simulink model "TBS_SIM_UDP_HIL"  (R2016b)
settings: Solver=ode5  StartTime=0.0  StopTime=inf  FixedStep=0.005  RelTol=1e-3  EnableMultiTasking=on
PreLoadFcn:
  | TBS_Cai_simu_init_20170316
StopFcn:
  | TBS_SIMULATION_LOG
undefined symbols (not defined in the file): air_density, L1X, L2X, L3X, L3Y, MAC1, MAC2, MAC3, magnitude, motor_m0, motor_t0, ORIGIN_CD, ORIGIN_CL, ORIGIN_CM, S_seg1, S_seg2, S_seg3, Standard_Devices, UDP_Protocol, y_ac
libraries: aerolibconvert2 x9, sldrtlib x4, aerolibwind2 x3, aerolibtransform2 x2, aerolib6dof2 x1, simulink x1, aerolibasang x1
settings Model: SimulationMode=external  Creator=SUN Jingxuan  LastModifiedBy=SUN Jingxuan
settings SolverCC: EnableConcurrentExecution=on
settings DataIOCC: LimitDataPoints=on  SaveFormat=StructureWithTime
settings OptimizationCC: BlockReduction=off  OptimizeBlockIOStorage=off  BufferReuse=off  GlobalBufferReuse=off  ExpressionFolding=off  LocalBlockOutputs=off
settings DebuggingCC: SFUnexpectedBacktrackingDiag=warning  SFNoUnconditionalDefaultTransitionDiag=warning  SFExecutionAtInitializationDiag=none
settings HardwareCC: TargetBitPerLong=64  TargetBitPerPointer=64  TargetIntDivRoundTo=Zero  TargetEndianess=LittleEndian  TargetWordSize=64  TargetHWDeviceType=Intel->x86-64
settings ModelReferenceCC: PropagateSignalLabelsOutOfModel=off
settings RTWCC: SystemTargetFile=sldrt.tlc  TemplateMakefile=sldrt.tmf  Description=Simulink Desktop Real-Time  RTWCompilerOptimization=on
settings CodeAppCC: MaxIdLength=95
settings SimulinkDesktopRealTimeCC: TargetPreCompLibLocation=E:\MATLAB2016\toolbox\sldrt\lib\win64  TargetLangStandard=C89/C90 (ANSI)  SupportVariableSizeSignals=off
settings ConfigComp: CovMetricSettings=dw  CovHtmlReporting=on  CovSaveCumulativeToWorkspaceVar=on  CovSaveSingleToWorkspaceVar=on  CovExternalEMLEnable=off

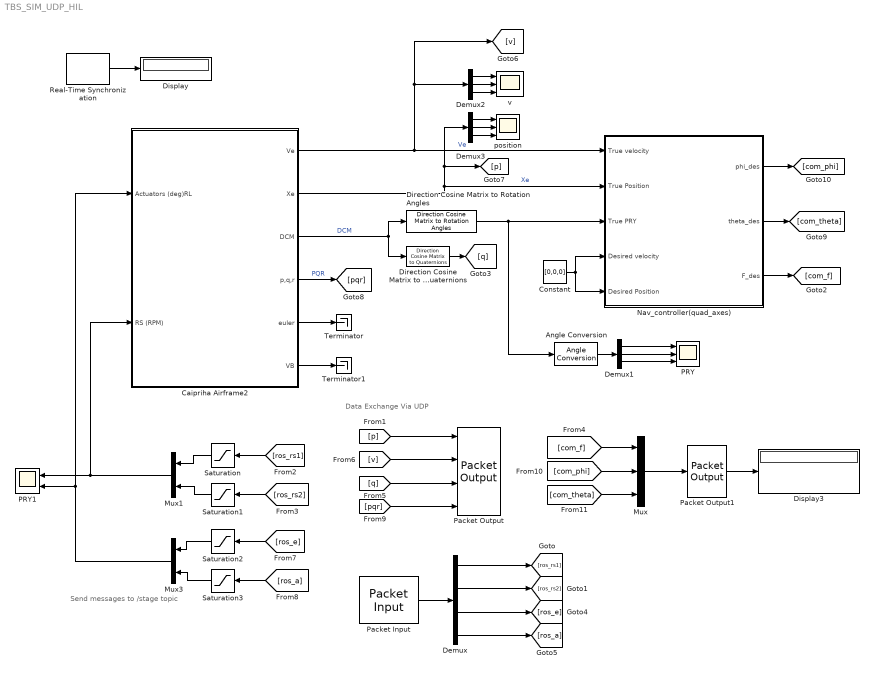
== system TBS_SIM_UDP_HIL ==
  note: Data Exchange Via UDP
  note: Send messages to /stage topic
  Angle Conversion : aerolibconvert2/Angle Conversion  IU=rad  OU=deg
  Caipriha Airframe2 : Subsystem
  Constant : Constant  Value=[0,0,0]
  Demux : Demux
  Demux1 : Demux  Outputs=3
  Demux2 : Demux  Outputs=3
  Demux3 : Demux  Outputs=3
  Direction Cosine Matrix to Rotation Angles : aerolibtransform2/Direction Cosine Matrix to Rotation Angles  rotationOrder=YZX  lim=Default
      settings: AttributesFormatString=Rotation Order: %<rotationOrder>
  Direction Cosine Matrix to Quaternions : aerolibtransform2/Direction Cosine Matrix  to Quaternions
  Display : Display
  Display3 : Display
  Mux : Mux  Inputs=3
  Mux1 : Mux  Inputs=2
  Mux3 : Mux  Inputs=2
  Nav_controller(quad_axes) : Subsystem
  PRY : Scope  NumInputPorts=3
  PRY1 : Scope  NumInputPorts=2
  Packet Input : sldrtlib/Packet Input  SampleTime=-1  MaxMissedTicks=10  ShowMissedTicks=off  YieldWhenWaiting=off  DrvName=Standard_Devices/UDP_Protocol  DrvAddress=49001  DrvOptions=[3232235791 49001]  PacketSize=32  DataTypes='4*double'  ShowReady=off  ShowError=off  PacketID=1  ByteOrder=1  ShowTimestamp=off
      settings: AttributesFormatString=Standard Devices\nUDP Protocol [BF69h]
  Packet Output : sldrtlib/Packet Output  SampleTime=-1  MaxMissedTicks=10  ShowMissedTicks=off  YieldWhenWaiting=off  DrvName=Standard_Devices/UDP_Protocol  DrvAddress=49005  DrvOptions=[3232235791 49000]  PacketSize=104  DataTypes={'3*double','3*double','4*double','3*double'}  ShowReady=off  ShowError=off  PacketID=1  ByteOrder=1  InitialValue=[0 0 0 0 0 0 0.7071 0 -0.7071 0 0 0 0]  FinalValue=[]
      settings: AttributesFormatString=Standard Devices\nUDP Protocol [BF6Dh]
  Packet Output1 : sldrtlib/Packet Output  SampleTime=-1  MaxMissedTicks=10  ShowMissedTicks=on  YieldWhenWaiting=off  DrvName=Standard_Devices/UDP_Protocol  DrvAddress=49006  DrvOptions=[3232235791 49005]  PacketSize=24  DataTypes='3*double'  ShowReady=off  ShowError=off  PacketID=1  ByteOrder=1  InitialValue=[8;0;0]  FinalValue=[]
      settings: AttributesFormatString=Standard Devices\nUDP Protocol [BF6Eh]
  Real-Time Synchronization : sldrtlib/Real-Time Synchronization  SampleTime=0.02  MaxMissedTicks=10  ShowMissedTicks=on  YieldWhenWaiting=off
  Saturation : Saturate  UpperLimit=10000  LowerLimit=0
  Saturation1 : Saturate  UpperLimit=10000  LowerLimit=0
  Saturation2 : Saturate  UpperLimit=16.5  LowerLimit=-23
  Saturation3 : Saturate  UpperLimit=16.5  LowerLimit=-23
  Terminator : Terminator
  Terminator1 : Terminator
  position : Scope  NumInputPorts=3
  "v " : Scope  NumInputPorts=3
  wires:
  Mux3/1 -> Caipriha Airframe2/1(Actuators (deg)RL), PRY1/2
  Mux1/1 -> Caipriha Airframe2/2(RS (RPM)), PRY1/1
  Constant/1 -> Nav_controller(quad_axes)/4(Desired velocity), Nav_controller(quad_axes)/5(Desired Position)
  Saturation/1 -> Mux1/1
  Saturation1/1 -> Mux1/2
  Saturation2/1 -> Mux3/1
  Saturation3/1 -> Mux3/2
  Demux2/1 -> "v "/1
  Demux2/2 -> "v "/2
  Demux2/3 -> "v "/3
  Caipriha Airframe2/1(Ve) -> [v], Demux2/1, Nav_controller(quad_axes)/1(True velocity)  "Ve"
  Demux3/1 -> position/1
  Demux3/2 -> position/2
  Demux3/3 -> position/3
  Caipriha Airframe2/2(Xe) -> Demux3/1, [p], Nav_controller(quad_axes)/2(True Position)  "Xe"
  Caipriha Airframe2/3(DCM) -> Direction Cosine Matrix to Rotation Angles/1, Direction Cosine Matrix to Quaternions/1  "DCM"
  Direction Cosine Matrix to Rotation Angles/1 -> Angle Conversion/1, Nav_controller(quad_axes)/3(True PRY)
  Demux1/1 -> PRY/1
  Demux1/2 -> PRY/2
  Demux1/3 -> PRY/3
  Angle Conversion/1 -> Demux1/1
  Nav_controller(quad_axes)/3(F_des) -> [com_f]
  Nav_controller(quad_axes)/2("theta_des ") -> [com_theta]
  Nav_controller(quad_axes)/1(phi_des) -> [com_phi]
  [ros_rs1] -> Saturation/1
  [ros_rs2] -> Saturation1/1
  [ros_e] -> Saturation2/1
  [ros_a] -> Saturation3/1
  Direction Cosine Matrix to Quaternions/1 -> [q]
  [p] -> Packet Output/1
  [pqr] -> Packet Output/4
  [v] -> Packet Output/2
  [q] -> Packet Output/3
  Packet Input/1 -> Demux/1
  Demux/1 -> [ros_rs1]
  Demux/2 -> [ros_rs2]
  Demux/3 -> [ros_e]
  Demux/4 -> [ros_a]
  Mux/1 -> Packet Output1/1
  Packet Output1/1 -> Display3/1
  Real-Time Synchronization/1 -> Display/1
  Caipriha Airframe2/4(p,q,r) -> [pqr]  "PQR"
  [com_f] -> Mux/1
  [com_phi] -> Mux/2
  [com_theta] -> Mux/3
  Caipriha Airframe2/5(euler) -> Terminator/1
  Caipriha Airframe2/6("VB ") -> Terminator1/1

== system TBS_SIM_UDP_HIL/Caipriha Airframe2 ==
  Actuators (deg)RL : Inport
  RS (RPM) : Inport  Port=2
  6DOF (Quaternion) : aerolib6dof2/6DOF (Euler Angles)  units=Metric (MKS)  mtype=Fixed  rep=Quaternion  xme_0=init_pos_hov  Vm_0=init_vel_hov  eul_0=init_att_hov  pm_0=[0 0 0]  mass_0=0.876  mass_e=0.5  mass_f=2.0  inertia=Inertia  inertia_e=eye(3)  inertia_f=2*eye(3)  k_quat=1.0  vre_flag=on
  Aerodynamic Coefficient : Subsystem
  Alpha,Beta,Mach : Subsystem  AncestorBlock=aeroblk_lib_HL20/HL20 Airframe/Alpha,Beta,Mach
  Angle Conversion : aerolibconvert2/Angle Conversion  IU=rad  OU=deg
  Constant2 : Constant  Value=8.541
  Display2 : Display
  Environment Models1 : Subsystem  AncestorBlock=aeroblk_lib_HL20/HL20 Airframe/Environment Models
  Force&Moments : Subsystem
  Scope : Scope
  Terminator1 : Terminator  Commented=on
  Terminator2 : Terminator  Commented=on
  "Thrust " : Subsystem
  Ve : Outport  InitialOutput=0
  Xe : Outport  Port=2  InitialOutput=0
  DCM : Outport  Port=3  InitialOutput=0
  p,q,r : Outport  Port=4  InitialOutput=0
  euler : Outport  Port=5  InitialOutput=0
  "VB " : Outport  Port=6  InitialOutput=0
  wires:
  6DOF (Quaternion)/5 -> "VB "/1, Alpha,Beta,Mach/2(Vb)
  6DOF (Quaternion)/1 -> Environment Models1/1(Ve), Ve/1
  Constant2/1 -> Force&Moments/5(Gravity)
  6DOF (Quaternion)/4 -> Environment Models1/3(DCM), DCM/1, Force&Moments/6(DCM)
  6DOF (Quaternion)/3 -> euler/1
  Alpha,Beta,Mach/3(V_aircraft) -> Aerodynamic Coefficient/4(V), "Thrust "/2("AS ")
  Alpha,Beta,Mach/2(Incid) -> Angle Conversion/1, Aerodynamic Coefficient/5(Incid)
  "Thrust "/2(MT1) -> Force&Moments/2(MT)
  "Thrust "/1(F_T) -> Force&Moments/1("FT ")
  "Thrust "/4(T2) -> Aerodynamic Coefficient/2(T2)
  "Thrust "/3(T1) -> Aerodynamic Coefficient/1("T1 ")
  Aerodynamic Coefficient/2(M) -> Force&Moments/4(M)
  Aerodynamic Coefficient/1(F) -> Force&Moments/3(F)
  RS (RPM)/1 -> "Thrust "/1(RS1)
  Actuators (deg)RL/1 -> Aerodynamic Coefficient/3(Actuators)
  Environment Models1/1(Wind Velocity) -> Alpha,Beta,Mach/1(Wind Velocity)
  6DOF (Quaternion)/7 -> Terminator2/1
  6DOF (Quaternion)/6 -> p,q,r/1
  6DOF (Quaternion)/2 -> Environment Models1/2(Position), Xe/1
  6DOF (Quaternion)/8 -> Terminator1/1
  Force&Moments/2(LMN) -> 6DOF (Quaternion)/2
  Force&Moments/1(X,Y,Z) -> 6DOF (Quaternion)/1
  Alpha,Beta,Mach/1("[Vb]_total") -> Aerodynamic Coefficient/6(Vb_total)
  Angle Conversion/1 -> Scope/1, Display2/1

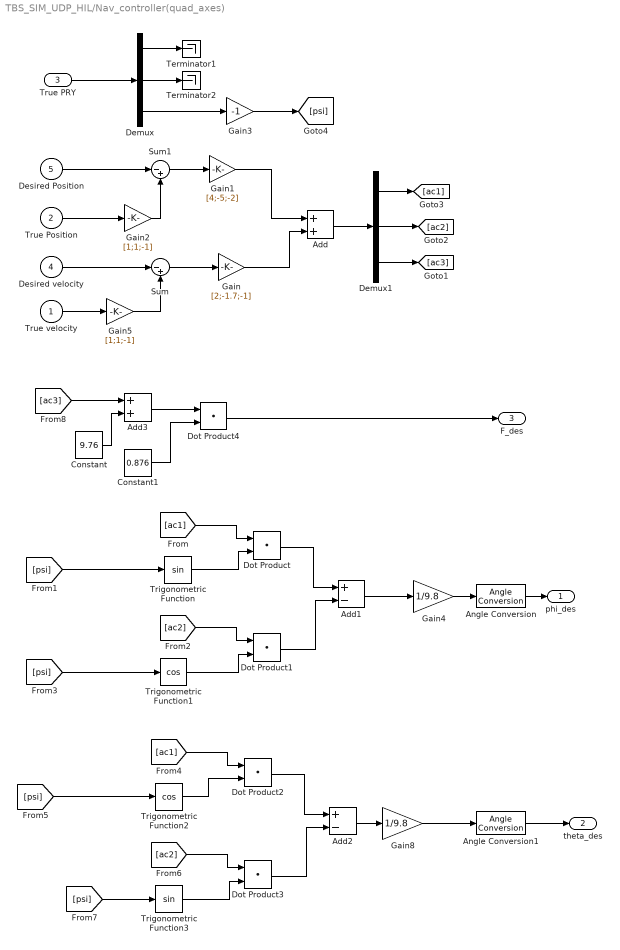
== system TBS_SIM_UDP_HIL/Nav_controller(quad_axes) ==
  True velocity : Inport
  True Position : Inport  Port=2
  True PRY : Inport  Port=3
  Desired velocity : Inport  Port=4
  Desired Position : Inport  Port=5
  Add : Sum
  Add1 : Sum  Inputs=+-
  Add2 : Sum  Inputs=+-
  Add3 : Sum
  Angle Conversion : aerolibconvert2/Angle Conversion  IU=rad  OU=deg
  Angle Conversion1 : aerolibconvert2/Angle Conversion  IU=rad  OU=deg
  Constant : Constant  Value=9.76
  Constant1 : Constant  Value=0.876
  Demux : Demux  Outputs=3
  Demux1 : Demux  Outputs=3
  Dot Product{,1..4} (5 alike) : DotProduct  InputSameDT=on  OutDataTypeStr=Inherit: Inherit via internal rule
  Gain : Gain  Gain=[2;-1.7;-1]
  Gain1 : Gain  Gain=[4;-5;-2]
  Gain2 : Gain  Gain=[1;1;-1]
  Gain3 : Gain  Gain=-1
  Gain4 : Gain  Gain=1/9.8
  Gain5 : Gain  Gain=[1;1;-1]
  Gain8 : Gain  Gain=1/9.8
  Sum : Sum  Inputs=|-+
  Sum1 : Sum  Inputs=|-+
  Terminator1 : Terminator
  Terminator2 : Terminator
  Trigonometric Function : Trigonometry
  Trigonometric Function1 : Trigonometry  Operator=cos
  Trigonometric Function2 : Trigonometry  Operator=cos
  Trigonometric Function3 : Trigonometry
  phi_des : Outport
  "theta_des " : Outport  Port=2
  F_des : Outport  Port=3
  wires:
  True velocity/1 -> Gain5/1
  Desired velocity/1 -> Sum/1
  Sum/1 -> Gain/1
  Sum1/1 -> Gain1/1
  Gain1/1 -> Add/1
  Gain/1 -> Add/2
  True PRY/1 -> Demux/1
  Demux/1 -> Terminator1/1
  Demux/3 -> Gain3/1
  Demux/2 -> Terminator2/1
  Add/1 -> Demux1/1
  Demux1/2 -> [ac2]
  [ac1] -> Dot Product/1
  Trigonometric Function/1 -> Dot Product/2
  [psi] -> Trigonometric Function/1
  [ac2] -> Dot Product1/1
  Trigonometric Function1/1 -> Dot Product1/2
  [psi] -> Trigonometric Function1/1
  Dot Product/1 -> Add1/1
  Dot Product1/1 -> Add1/2
  Add1/1 -> Gain4/1
  [ac1] -> Dot Product2/1
  Trigonometric Function2/1 -> Dot Product2/2
  [psi] -> Trigonometric Function2/1
  [ac2] -> Dot Product3/1
  Trigonometric Function3/1 -> Dot Product3/2
  [psi] -> Trigonometric Function3/1
  Dot Product2/1 -> Add2/1
  Dot Product3/1 -> Add2/2
  Add2/1 -> Gain8/1
  [ac3] -> Add3/1
  Constant/1 -> Add3/2
  Add3/1 -> Dot Product4/1
  Constant1/1 -> Dot Product4/2
  Dot Product4/1 -> F_des/1
  Demux1/1 -> [ac1]
  Demux1/3 -> [ac3]
  True Position/1 -> Gain2/1
  Gain2/1 -> Sum1/2
  Desired Position/1 -> Sum1/1
  Gain3/1 -> [psi]
  Gain4/1 -> Angle Conversion/1
  Angle Conversion/1 -> phi_des/1
  Gain8/1 -> Angle Conversion1/1
  Angle Conversion1/1 -> "theta_des "/1
  Gain5/1 -> Sum/2

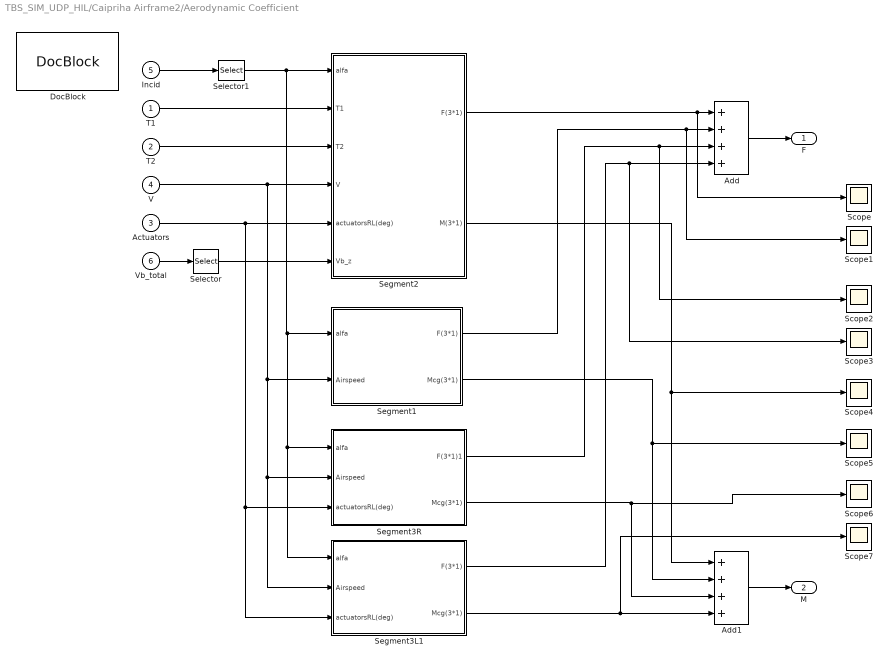
== system TBS_SIM_UDP_HIL/Caipriha Airframe2/Aerodynamic Coefficient ==
  "T1 " : Inport
  T2 : Inport  Port=2
  Actuators : Inport  Port=3
  V : Inport  Port=4
  Incid : Inport  Port=5
  Vb_total : Inport  Port=6
  Add : Sum  Inputs=++++
  Add1 : Sum  Inputs=++++
  DocBlock : simulink/Model-Wide Utilities/DocBlock  DocumentType=Text
      content=|
      | Segment definition: F:\MATLAB\TBS dynamic\segment.png
  Scope{,1..7} (8 alike) : Scope
  Segment1 : Subsystem
  Segment2 : Subsystem
  Segment3L1 : Subsystem
  Segment3R : Subsystem
  Selector : Selector  InputPortWidth=3  IndexOptions=Index vector (dialog)  Indices=[3]  OutputSizes=1
  Selector1 : Selector  InputPortWidth=2  IndexOptions=Index vector (dialog)  Indices=[1]  OutputSizes=1
  F : Outport
  M : Outport  Port=2
  wires:
  T2/1 -> Segment2/3(T2)
  "T1 "/1 -> Segment2/2("T1 ")
  Selector1/1 -> Segment3L1/1(alfa), Segment3R/1(alfa), Segment1/1(alfa), Segment2/1(alfa)
  Incid/1 -> Selector1/1
  Actuators/1 -> Segment3L1/3("actuatorsRL(deg) "), Segment3R/3("actuatorsRL(deg) "), Segment2/5("actuatorsRL(deg) ")
  V/1 -> Segment3L1/2(Airspeed), Segment3R/2(Airspeed), Segment1/2(Airspeed), Segment2/4(V)
  Selector/1 -> Segment2/6(Vb_z)
  Vb_total/1 -> Selector/1
  Segment2/1(F(3*1)) -> Scope/1, Add/1
  Segment1/1(F(3*1)) -> Scope1/1, Add/2
  Segment3R/1(F(3*1)1) -> Add/3, Scope2/1
  Segment3L1/1(F(3*1)) -> Scope3/1, Add/4
  Add/1 -> F/1
  Add1/1 -> M/1
  Segment2/2(M(3*1)) -> Scope4/1, Add1/1
  Segment1/2(Mcg(3*1)) -> Add1/2, Scope5/1
  Segment3R/2(Mcg(3*1)) -> Scope6/1, Add1/3
  Segment3L1/2(Mcg(3*1)) -> Scope7/1, Add1/4

== system TBS_SIM_UDP_HIL/Caipriha Airframe2/Alpha,Beta,Mach ==
  Wind Velocity : Inport  PortDimensions=3
  Vb : Inport  Port=2  PortDimensions=3
  "Incidence, Sideslip & Airspeed" : aerolibasang/Incidence, Sideslip, & Airspeed
  Mux : Mux  Inputs=2
  Sum : Sum  Inputs=|+-  SaturateOnIntegerOverflow=on  InputSameDT=on  OutDataTypeStr=Inherit: Same as first input
  "[Vb]_total" : Outport
  Incid : Outport  Port=2
  V_aircraft : Outport  Port=3
  wires:
  Sum/1 -> "[Vb]_total"/1, "Incidence, Sideslip & Airspeed"/1
  Wind Velocity/1 -> Sum/2
  "Incidence, Sideslip & Airspeed"/1 -> Mux/1  "Alpha"
  Mux/1 -> Incid/1
  "Incidence, Sideslip & Airspeed"/2 -> Mux/2  "Beta"
  Vb/1 -> Sum/1
  "Incidence, Sideslip & Airspeed"/3 -> V_aircraft/1

== system TBS_SIM_UDP_HIL/Caipriha Airframe2/Environment Models1 ==
  Ve : Inport
  Position : Inport  Port=2
  DCM : Inport  Port=3
  Abs : Abs
  Discrete Wind Gust Model : aerolibwind2/Discrete Wind Gust Model  units=Metric (MKS)  Gx=on  Gy=on  Gz=on  t_0=30  d_m=[100 100 100]  v_m=[1 1 1]
  Dot Product : DotProduct  SaturateOnIntegerOverflow=on  OutDataTypeStr=Inherit: Inherit via internal rule
  Horizontal Wind Model1 : aerolibwind2/Horizontal Wind Model  units=Metric (MKS)  Vw_source=Internal  Vwind=1  W_source=Internal  Wdeg=83
  Scope2 : Scope
  Selector : Selector  InputPortWidth=3  IndexOptions=Index vector (dialog)  Indices=[3]  OutputSizes=1
  Sum : Sum  Inputs=+++
  V : Math  Operator=sqrt  SaturateOnIntegerOverflow=on
  Wind Shear Model : aerolibwind2/Wind Shear Model  units=Metric (MKS)  phase=Other  W_20=0  Wdeg=0
  Wind Velocity : Outport  InitialOutput=0
  wires:
  V/1 -> Discrete Wind Gust Model/1
  Dot Product/1 -> V/1
  Ve/1 -> Dot Product/2, Dot Product/1
  Position/1 -> Selector/1
  Selector/1 -> Abs/1
  Abs/1 -> Wind Shear Model/1
  DCM/1 -> Horizontal Wind Model1/1, Wind Shear Model/2
  Wind Shear Model/1 -> Sum/2
  Discrete Wind Gust Model/1 -> Sum/1
  Sum/1 -> Scope2/1, Wind Velocity/1
  Horizontal Wind Model1/1 -> Sum/3

== system TBS_SIM_UDP_HIL/Caipriha Airframe2/Force&Moments ==
  "FT " : Inport
  MT : Inport  Port=2
  F : Inport  Port=3
  M : Inport  Port=4
  Gravity : Inport  Port=5
  DCM : Inport  Port=6
  Constant1 : Constant  Value=0
  Mux : Mux  Inputs=3
  Product : Product  Multiplication=Matrix(*)
  Sum : Sum  SaturateOnIntegerOverflow=on  InputSameDT=on  OutDataTypeStr=Inherit: Same as first input
  Sum1 : Sum
  Sum2 : Sum  Inputs=|++  SaturateOnIntegerOverflow=on  InputSameDT=on  OutDataTypeStr=Inherit: Same as first input
  X,Y,Z : Outport  InitialOutput=0
  LMN : Outport  Port=2  InitialOutput=0
  wires:
  Mux/1 -> Product/2
  Constant1/1 -> Mux/1, Mux/2
  Gravity/1 -> Mux/3
  DCM/1 -> Product/1
  Product/1 -> Sum2/2
  Sum2/1 -> X,Y,Z/1
  Sum/1 -> Sum2/1
  MT/1 -> Sum1/2
  "FT "/1 -> Sum/2
  Sum1/1 -> LMN/1
  M/1 -> Sum1/1
  F/1 -> Sum/1

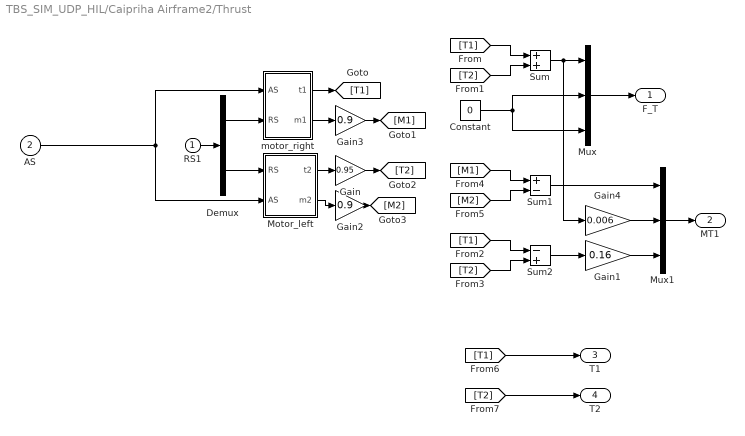
== system TBS_SIM_UDP_HIL/Caipriha Airframe2/Thrust  ==
  RS1 : Inport
  "AS " : Inport  Port=2
  Constant : Constant  Value=0
  Demux : Demux  Outputs=2
  Gain : Gain  Gain=0.95
  Gain1 : Gain  Gain=0.16
  Gain2 : Gain  Gain=0.9
  Gain3 : Gain  Gain=0.9
  Gain4 : Gain  Gain=0.006
  Motor_left : Subsystem
  Mux : Mux  Inputs=3
  Mux1 : Mux  Inputs=3
  Sum : Sum
  Sum1 : Sum  Inputs=+-
  Sum2 : Sum  Inputs=-+
  motor_right : Subsystem
  F_T : Outport
  MT1 : Outport  Port=2
  T1 : Outport  Port=3
  T2 : Outport  Port=4
  wires:
  Motor_left/2("m2 ") -> Gain2/1
  Gain3/1 -> [M1]
  Gain2/1 -> [M2]
  Gain/1 -> [T2]
  Motor_left/1(t2) -> Gain/1
  "AS "/1 -> Motor_left/2(AS), motor_right/1(AS)
  [T2] -> T2/1
  [T1] -> T1/1
  Gain4/1 -> Mux1/2
  [M2] -> Sum1/2
  [M1] -> Sum1/1
  [T2] -> Sum2/2
  [T1] -> Sum2/1
  [T2] -> Sum/2
  [T1] -> Sum/1
  motor_right/2("m1 ") -> Gain3/1
  motor_right/1(t1) -> [T1]
  Constant/1 -> Mux/2, Mux/3
  Sum1/1 -> Mux1/1
  Gain1/1 -> Mux1/3
  Sum2/1 -> Gain1/1
  Sum/1 -> Gain4/1, Mux/1
  Mux1/1 -> MT1/1
  Mux/1 -> F_T/1
  Demux/2 -> Motor_left/1(RS)
  Demux/1 -> motor_right/2(RS)
  RS1/1 -> Demux/1

== system TBS_SIM_UDP_HIL/Caipriha Airframe2/Aerodynamic Coefficient/Segment1 ==
  alfa : Inport
  Airspeed : Inport  Port=2
  Add5 : Sum  Inputs=++|
  Constant1 : Constant  Value=0
  Constant2 : Constant  Value=0
  Constant3 : Constant  Value=0
  Gain11 : Gain  Gain=L1X
  Gain3 : Gain  Gain=-1
  Gain4 : Gain  Gain=-1
  Mux : Mux  Inputs=3
  Mux1 : Mux  Inputs=3
  right wing : Subsystem
  F(3*1) : Outport
  Mcg(3*1) : Outport  Port=2
  wires:
  Airspeed/1 -> right wing/1(v)
  Mux1/1 -> Mcg(3*1)/1
  Constant3/1 -> Mux1/3
  Add5/1 -> Mux1/2
  Mux/1 -> F(3*1)/1
  Constant1/1 -> Mux/2
  Gain3/1 -> Mux/3
  Gain4/1 -> Mux/1
  right wing/2(Fx) -> Gain4/1
  right wing/1(Fz) -> Gain3/1, Gain11/1
  Gain11/1 -> Add5/1
  right wing/3(Mac) -> Add5/2
  Constant2/1 -> Mux1/1
  alfa/1 -> right wing/2("ALFA ")

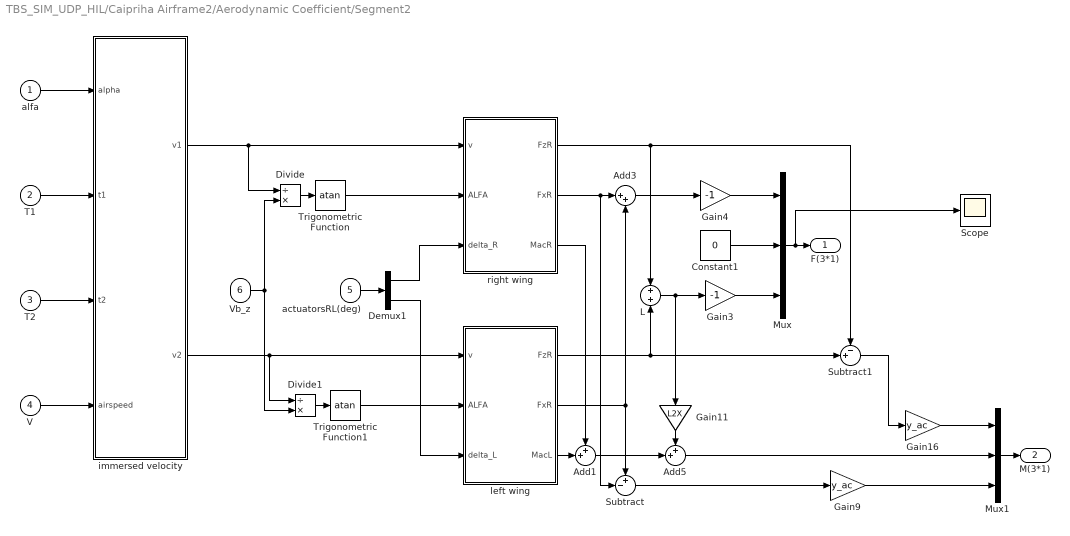
== system TBS_SIM_UDP_HIL/Caipriha Airframe2/Aerodynamic Coefficient/Segment2 ==
  alfa : Inport
  "T1 " : Inport  Port=2
  T2 : Inport  Port=3
  V : Inport  Port=4
  "actuatorsRL(deg) " : Inport  Port=5
  Vb_z : Inport  Port=6
  Add1 : Sum  Inputs=++|
  Add3 : Sum  Inputs=|++
  Add5 : Sum  Inputs=++|
  Constant1 : Constant  Value=0
  Demux1 : Demux  Outputs=2
  Divide : Product  Inputs=/*
  Divide1 : Product  Inputs=/*
  Gain11 : Gain  Gain=L2X
  Gain16 : Gain  Gain=y_ac
  Gain3 : Gain  Gain=-1
  Gain4 : Gain  Gain=-1
  Gain9 : Gain  Gain=y_ac
  L : Sum
  Mux : Mux  Inputs=3
  Mux1 : Mux  Inputs=3
  Scope : Scope
  Subtract : Sum  Inputs=+-|
  Subtract1 : Sum  Inputs=-+|
  Trigonometric Function : Trigonometry  Operator=atan  OutputSignalType=real
  Trigonometric Function1 : Trigonometry  Operator=atan
  immersed velocity : Subsystem
  left wing : Subsystem
  right wing : Subsystem
  F(3*1) : Outport
  M(3*1) : Outport  Port=2
  wires:
  V/1 -> immersed velocity/4(airspeed)
  immersed velocity/2(v2) -> left wing/1(v), Divide1/1
  immersed velocity/1(v1) -> right wing/1(v), Divide/1
  Mux1/1 -> M(3*1)/1
  Gain9/1 -> Mux1/3
  Add5/1 -> Mux1/2
  Subtract/1 -> Gain9/1
  Mux/1 -> Scope/1, F(3*1)/1
  Constant1/1 -> Mux/2
  Gain3/1 -> Mux/3
  Gain4/1 -> Mux/1
  Add3/1 -> Gain4/1
  L/1 -> Gain3/1, Gain11/1
  "actuatorsRL(deg) "/1 -> Demux1/1
  right wing/2(FxR) -> Subtract/2, Add3/1
  right wing/1(FzR) -> Subtract1/1, L/1
  T2/1 -> immersed velocity/3(t2)
  "T1 "/1 -> immersed velocity/2("t1 ")
  Vb_z/1 -> Divide1/2, Divide/2
  Divide/1 -> Trigonometric Function/1
  Divide1/1 -> Trigonometric Function1/1
  alfa/1 -> immersed velocity/1(alpha)
  left wing/2(FxR) -> Add3/2, Subtract/1
  left wing/3(MacL) -> Add1/2
  right wing/3(MacR) -> Add1/1
  left wing/1(FzR) -> Subtract1/2, L/2
  Gain11/1 -> Add5/1
  Add1/1 -> Add5/2
  Subtract1/1 -> Gain16/1
  Gain16/1 -> Mux1/1
  Demux1/1 -> right wing/3(delta_R)
  Demux1/2 -> left wing/3(delta_L)
  Trigonometric Function/1 -> right wing/2("ALFA ")
  Trigonometric Function1/1 -> left wing/2("ALFA ")

== system TBS_SIM_UDP_HIL/Caipriha Airframe2/Aerodynamic Coefficient/Segment3L1 ==
  alfa : Inport
  Airspeed : Inport  Port=2
  "actuatorsRL(deg) " : Inport  Port=3
  Constant1 : Constant  Value=0
  Gain1 : Gain  Gain=L3X
  Gain2 : Gain  Gain=-L3Y
  Gain3 : Gain  Gain=-1
  Gain4 : Gain  Gain=-1
  Gain5 : Gain  Gain=L3Y
  Mux : Mux  Inputs=3
  Mux1 : Mux  Inputs=3
  Selector : Selector  InputPortWidth=2  IndexOptions=Index vector (dialog)  Indices=[2]  OutputSizes=1
  Sum : Sum  Inputs=++|
  wing : Subsystem
  F(3*1) : Outport
  Mcg(3*1) : Outport  Port=2
  wires:
  Airspeed/1 -> wing/1(v)
  Mux1/1 -> Mcg(3*1)/1
  Gain2/1 -> Mux1/3
  wing/3(Mac) -> Sum/2
  Mux/1 -> F(3*1)/1
  Constant1/1 -> Mux/2
  Gain3/1 -> Mux/3
  Gain4/1 -> Mux/1
  wing/2(Fx) -> Gain2/1, Gain4/1
  wing/1(Fz) -> Gain1/1, Gain3/1, Gain5/1
  "actuatorsRL(deg) "/1 -> Selector/1
  Gain5/1 -> Mux1/1
  Selector/1 -> wing/3(delta_R)
  alfa/1 -> wing/2("ALFA ")
  Sum/1 -> Mux1/2
  Gain1/1 -> Sum/1

== system TBS_SIM_UDP_HIL/Caipriha Airframe2/Aerodynamic Coefficient/Segment3R ==
  alfa : Inport
  Airspeed : Inport  Port=2
  "actuatorsRL(deg) " : Inport  Port=3
  Constant4 : Constant  Value=0
  Gain1 : Gain  Gain=L3X
  Gain2 : Gain  Gain=L3Y
  Gain5 : Gain  Gain=-1
  Gain6 : Gain  Gain=-1
  Gain7 : Gain  Gain=-L3Y
  Mux2 : Mux  Inputs=3
  Mux3 : Mux  Inputs=3
  Selector : Selector  InputPortWidth=2  IndexOptions=Index vector (dialog)  Indices=[1]  OutputSizes=1
  Sum : Sum  Inputs=++|
  right wing : Subsystem
  F(3*1)1 : Outport
  Mcg(3*1) : Outport  Port=2
  wires:
  Airspeed/1 -> right wing/1(v)
  "actuatorsRL(deg) "/1 -> Selector/1
  Selector/1 -> right wing/3(delta_R)
  alfa/1 -> right wing/2("ALFA ")
  Mux3/1 -> Mcg(3*1)/1
  Gain2/1 -> Mux3/3
  right wing/3(MacR) -> Sum/2
  Mux2/1 -> F(3*1)1/1
  Constant4/1 -> Mux2/2
  Gain5/1 -> Mux2/3
  Gain6/1 -> Mux2/1
  right wing/2(FxR) -> Gain2/1, Gain6/1
  right wing/1(FzR) -> Gain1/1, Gain5/1, Gain7/1
  Gain7/1 -> Mux3/1
  Sum/1 -> Mux3/2
  Gain1/1 -> Sum/1

== system TBS_SIM_UDP_HIL/Caipriha Airframe2/Thrust /Motor_left ==
  RS : Inport
  AS : Inport  Port=2
  As_Prelookup : PreLookup  BreakpointsData=AS_R  ExtrapMethod=Linear
  M1LOOKUP1 : Interpolation_n-D  Table=motor_m0'  InternalRulePriority=Speed
  RS_Prelookup1 : PreLookup  BreakpointsData=RS  ExtrapMethod=Linear
  T1LOOKUP : Interpolation_n-D  Table=motor_t0'  InternalRulePriority=Speed
  t2 : Outport
  "m2 " : Outport  Port=2
  wires:
  RS/1 -> RS_Prelookup1/1
  AS/1 -> As_Prelookup/1
  M1LOOKUP1/1 -> "m2 "/1
  T1LOOKUP/1 -> t2/1
  RS_Prelookup1/2 -> T1LOOKUP/4, M1LOOKUP1/4
  RS_Prelookup1/1 -> M1LOOKUP1/3, T1LOOKUP/3
  As_Prelookup/2 -> T1LOOKUP/2, M1LOOKUP1/2
  As_Prelookup/1 -> T1LOOKUP/1, M1LOOKUP1/1

== system TBS_SIM_UDP_HIL/Caipriha Airframe2/Thrust /motor_right ==
  AS : Inport
  RS : Inport  Port=2
  As_Prelookup : PreLookup  BreakpointsData=AS_R  ExtrapMethod=Linear
  M1LOOKUP1 : Interpolation_n-D  Table=motor_m0'  InternalRulePriority=Speed
  RS_Prelookup1 : PreLookup  BreakpointsData=RS  ExtrapMethod=Linear
  T1LOOKUP : Interpolation_n-D  Table=motor_t0'  InternalRulePriority=Speed
  t1 : Outport
  "m1 " : Outport  Port=2
  wires:
  M1LOOKUP1/1 -> "m1 "/1
  T1LOOKUP/1 -> t1/1
  RS_Prelookup1/2 -> T1LOOKUP/4, M1LOOKUP1/4
  RS_Prelookup1/1 -> T1LOOKUP/3, M1LOOKUP1/3
  As_Prelookup/2 -> T1LOOKUP/2, M1LOOKUP1/2
  As_Prelookup/1 -> T1LOOKUP/1, M1LOOKUP1/1
  RS/1 -> RS_Prelookup1/1
  AS/1 -> As_Prelookup/1

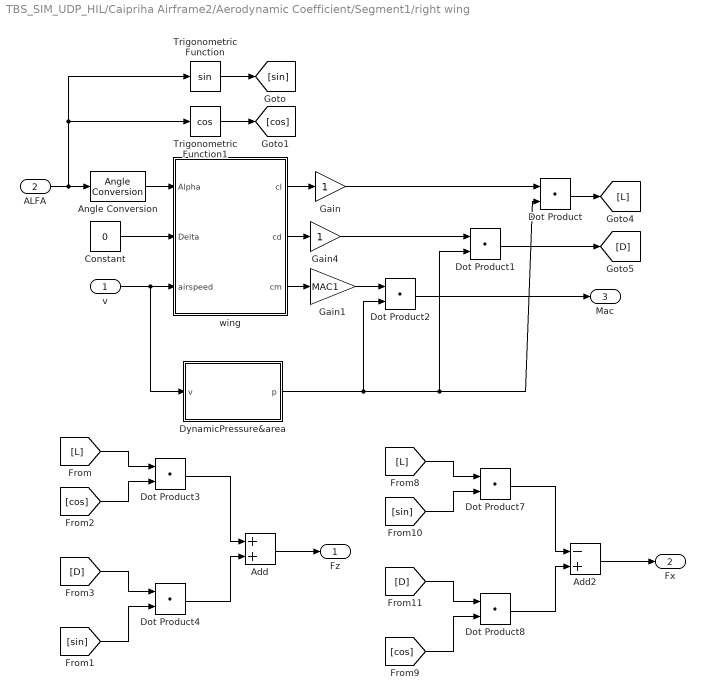
== system TBS_SIM_UDP_HIL/Caipriha Airframe2/Aerodynamic Coefficient/Segment1/right wing ==
  v : Inport
  "ALFA " : Inport  Port=2
  Add : Sum
  Add2 : Sum  Inputs=-+
  Angle Conversion : aerolibconvert2/Angle Conversion  IU=rad  OU=deg
  Constant : Constant  Value=0
  Dot Product{,1..4,7..8} (7 alike) : DotProduct  InputSameDT=on  OutDataTypeStr=Inherit: Inherit via internal rule
  DynamicPressure&area : Subsystem
  Gain : Gain
  Gain1 : Gain  Gain=MAC1
  Gain4 : Gain
  Trigonometric Function : Trigonometry
  Trigonometric Function1 : Trigonometry  Operator=cos
  wing : Subsystem
  Fz : Outport
  Fx : Outport  Port=2
  Mac : Outport  Port=3
  wires:
  wing/3(cm) -> Gain1/1
  Gain4/1 -> Dot Product1/1
  Gain/1 -> Dot Product/1
  wing/1(cl) -> Gain/1
  v/1 -> DynamicPressure&area/1(v), wing/3(airspeed)
  Constant/1 -> wing/2(Delta)
  DynamicPressure&area/1(p) -> Dot Product/2, Dot Product1/2, Dot Product2/2
  wing/2(cd) -> Gain4/1
  Gain1/1 -> Dot Product2/1
  Dot Product2/1 -> Mac/1
  Angle Conversion/1 -> wing/1(Alpha)
  Trigonometric Function/1 -> [sin]
  "ALFA "/1 -> Trigonometric Function/1, Trigonometric Function1/1, Angle Conversion/1
  Trigonometric Function1/1 -> [cos]
  Dot Product/1 -> [L]
  Dot Product1/1 -> [D]
  [L] -> Dot Product3/1
  [cos] -> Dot Product3/2
  [D] -> Dot Product4/1
  [sin] -> Dot Product4/2
  Dot Product3/1 -> Add/1
  Dot Product4/1 -> Add/2
  Add/1 -> Fz/1
  [L] -> Dot Product7/1
  [sin] -> Dot Product7/2
  [D] -> Dot Product8/1
  [cos] -> Dot Product8/2
  Dot Product7/1 -> Add2/1
  Dot Product8/1 -> Add2/2
  Add2/1 -> Fx/1

== system TBS_SIM_UDP_HIL/Caipriha Airframe2/Aerodynamic Coefficient/Segment2/immersed velocity ==
  alpha : Inport
  "t1 " : Inport  Port=2
  t2 : Inport  Port=3
  airspeed : Inport  Port=4
  "Immersed velocity " : Subsystem
  Immersed velocity 1 : Subsystem
  v1 : Outport
  v2 : Outport  Port=2
  wires:
  airspeed/1 -> "Immersed velocity "/2(airspeed), Immersed velocity 1/2(airspeed)
  alpha/1 -> Immersed velocity 1/3(alfa), "Immersed velocity "/3(alfa)
  Immersed velocity 1/1(v) -> v2/1
  "Immersed velocity "/1(v) -> v1/1
  t2/1 -> Immersed velocity 1/1(T)
  "t1 "/1 -> "Immersed velocity "/1(T)

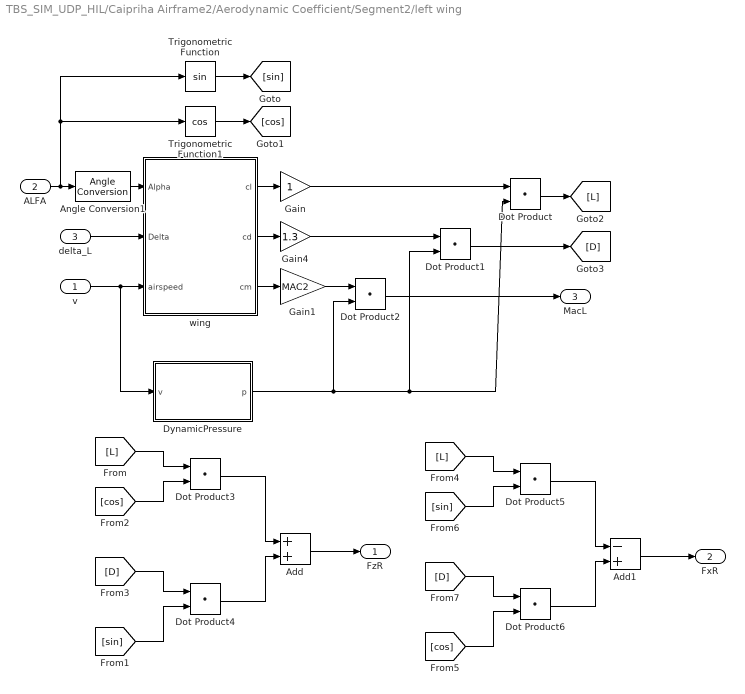
== system TBS_SIM_UDP_HIL/Caipriha Airframe2/Aerodynamic Coefficient/Segment2/left wing ==
  v : Inport
  "ALFA " : Inport  Port=2
  delta_L : Inport  Port=3
  Add : Sum
  Add1 : Sum  Inputs=-+
  Angle Conversion1 : aerolibconvert2/Angle Conversion  IU=rad  OU=deg
  Dot Product{,1..6} (7 alike) : DotProduct  InputSameDT=on  OutDataTypeStr=Inherit: Inherit via internal rule
  DynamicPressure : Subsystem
  Gain : Gain
  Gain1 : Gain  Gain=MAC2
  Gain4 : Gain  Gain=1.3
  Trigonometric Function : Trigonometry
  Trigonometric Function1 : Trigonometry  Operator=cos
  wing : Subsystem
  FzR : Outport
  FxR : Outport  Port=2
  MacL : Outport  Port=3
  wires:
  wing/3(cm) -> Gain1/1
  Gain4/1 -> Dot Product1/1
  Gain/1 -> Dot Product/1
  wing/1(cl) -> Gain/1
  v/1 -> DynamicPressure/1(v), wing/3(airspeed)
  delta_L/1 -> wing/2(Delta)
  DynamicPressure/1(p) -> Dot Product/2, Dot Product1/2, Dot Product2/2
  wing/2(cd) -> Gain4/1
  Gain1/1 -> Dot Product2/1
  Dot Product2/1 -> MacL/1
  Angle Conversion1/1 -> wing/1(Alpha)
  Trigonometric Function/1 -> [sin]
  "ALFA "/1 -> Trigonometric Function/1, Trigonometric Function1/1, Angle Conversion1/1
  Trigonometric Function1/1 -> [cos]
  Dot Product/1 -> [L]
  Dot Product1/1 -> [D]
  [L] -> Dot Product3/1
  [cos] -> Dot Product3/2
  [D] -> Dot Product4/1
  [sin] -> Dot Product4/2
  Dot Product3/1 -> Add/1
  Dot Product4/1 -> Add/2
  Add/1 -> FzR/1
  [L] -> Dot Product5/1
  [sin] -> Dot Product5/2
  [D] -> Dot Product6/1
  [cos] -> Dot Product6/2
  Dot Product5/1 -> Add1/1
  Dot Product6/1 -> Add1/2
  Add1/1 -> FxR/1

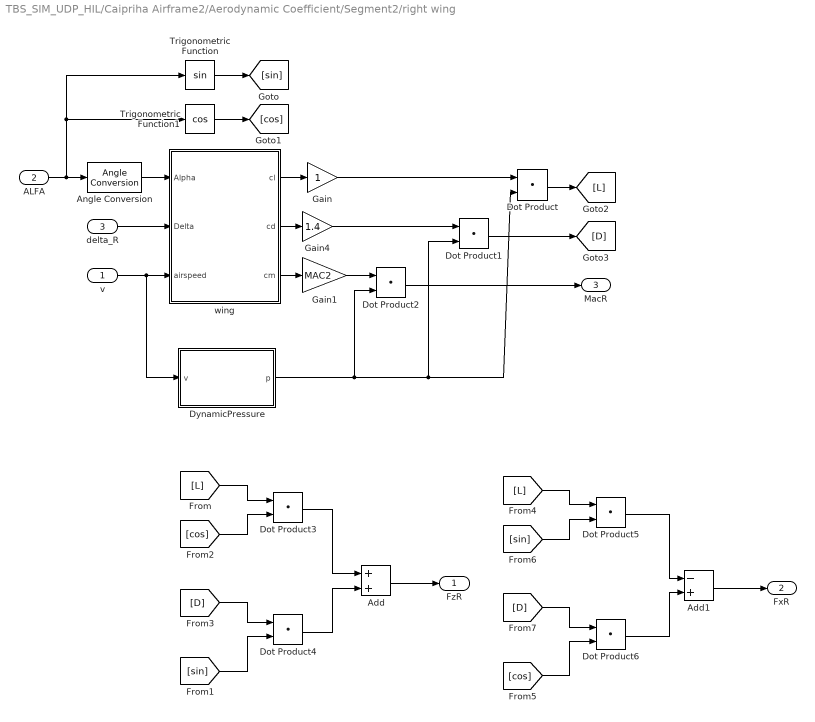
== system TBS_SIM_UDP_HIL/Caipriha Airframe2/Aerodynamic Coefficient/Segment2/right wing ==
  v : Inport
  "ALFA " : Inport  Port=2
  delta_R : Inport  Port=3
  Add : Sum
  Add1 : Sum  Inputs=-+
  Angle Conversion : aerolibconvert2/Angle Conversion  IU=rad  OU=deg
  Dot Product{,1..6} (7 alike) : DotProduct  InputSameDT=on  OutDataTypeStr=Inherit: Inherit via internal rule
  DynamicPressure : Subsystem
  Gain : Gain
  Gain1 : Gain  Gain=MAC2
  Gain4 : Gain  Gain=1.4
  Trigonometric Function : Trigonometry
  Trigonometric Function1 : Trigonometry  Operator=cos
  wing : Subsystem
  FzR : Outport
  FxR : Outport  Port=2
  MacR : Outport  Port=3
  wires:
  wing/3(cm) -> Gain1/1
  Gain4/1 -> Dot Product1/1
  Gain/1 -> Dot Product/1
  wing/1(cl) -> Gain/1
  v/1 -> DynamicPressure/1(v), wing/3(airspeed)
  delta_R/1 -> wing/2(Delta)
  DynamicPressure/1(p) -> Dot Product/2, Dot Product1/2, Dot Product2/2
  wing/2(cd) -> Gain4/1
  Gain1/1 -> Dot Product2/1
  Dot Product2/1 -> MacR/1
  Angle Conversion/1 -> wing/1(Alpha)
  Trigonometric Function/1 -> [sin]
  "ALFA "/1 -> Trigonometric Function/1, Trigonometric Function1/1, Angle Conversion/1
  Trigonometric Function1/1 -> [cos]
  Dot Product/1 -> [L]
  Dot Product1/1 -> [D]
  [L] -> Dot Product3/1
  [cos] -> Dot Product3/2
  [D] -> Dot Product4/1
  [sin] -> Dot Product4/2
  Dot Product3/1 -> Add/1
  Dot Product4/1 -> Add/2
  Add/1 -> FzR/1
  [L] -> Dot Product5/1
  [sin] -> Dot Product5/2
  [D] -> Dot Product6/1
  [cos] -> Dot Product6/2
  Dot Product5/1 -> Add1/1
  Dot Product6/1 -> Add1/2
  Add1/1 -> FxR/1

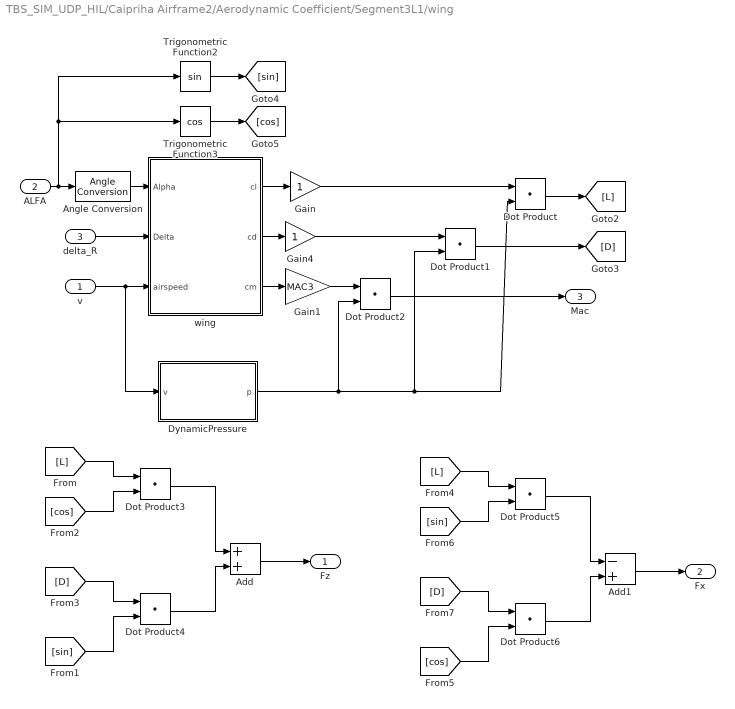
== system TBS_SIM_UDP_HIL/Caipriha Airframe2/Aerodynamic Coefficient/Segment3L1/wing ==
  v : Inport
  "ALFA " : Inport  Port=2
  delta_R : Inport  Port=3
  Add : Sum
  Add1 : Sum  Inputs=-+
  Angle Conversion : aerolibconvert2/Angle Conversion  IU=rad  OU=deg
  Dot Product{,1..6} (7 alike) : DotProduct  InputSameDT=on  OutDataTypeStr=Inherit: Inherit via internal rule
  DynamicPressure : Subsystem
  Gain : Gain
  Gain1 : Gain  Gain=MAC3
  Gain4 : Gain
  Trigonometric Function2 : Trigonometry
  Trigonometric Function3 : Trigonometry  Operator=cos
  wing : Subsystem
  Fz : Outport
  Fx : Outport  Port=2
  Mac : Outport  Port=3
  wires:
  wing/3(cm) -> Gain1/1
  Gain4/1 -> Dot Product1/1
  Gain/1 -> Dot Product/1
  wing/1(cl) -> Gain/1
  v/1 -> DynamicPressure/1(v), wing/3(airspeed)
  delta_R/1 -> wing/2(Delta)
  DynamicPressure/1(p) -> Dot Product/2, Dot Product1/2, Dot Product2/2
  wing/2(cd) -> Gain4/1
  Gain1/1 -> Dot Product2/1
  Dot Product2/1 -> Mac/1
  Angle Conversion/1 -> wing/1(Alpha)
  Trigonometric Function2/1 -> [sin]
  "ALFA "/1 -> Trigonometric Function2/1, Trigonometric Function3/1, Angle Conversion/1
  Trigonometric Function3/1 -> [cos]
  Dot Product/1 -> [L]
  Dot Product1/1 -> [D]
  [L] -> Dot Product3/1
  [cos] -> Dot Product3/2
  [D] -> Dot Product4/1
  [sin] -> Dot Product4/2
  Dot Product3/1 -> Add/1
  Dot Product4/1 -> Add/2
  Add/1 -> Fz/1
  [L] -> Dot Product5/1
  [sin] -> Dot Product5/2
  [D] -> Dot Product6/1
  [cos] -> Dot Product6/2
  Dot Product5/1 -> Add1/1
  Dot Product6/1 -> Add1/2
  Add1/1 -> Fx/1

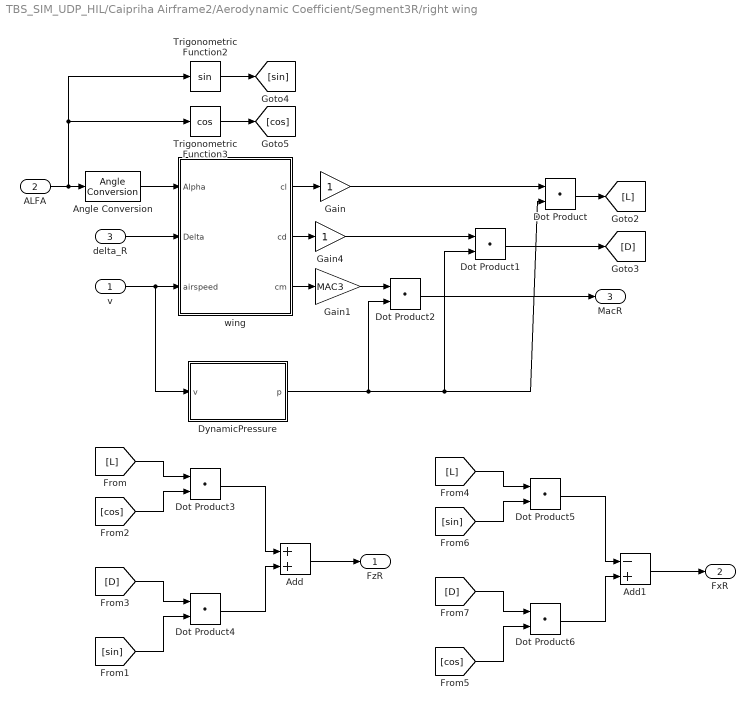
== system TBS_SIM_UDP_HIL/Caipriha Airframe2/Aerodynamic Coefficient/Segment3R/right wing ==
  v : Inport
  "ALFA " : Inport  Port=2
  delta_R : Inport  Port=3
  Add : Sum
  Add1 : Sum  Inputs=-+
  Angle Conversion : aerolibconvert2/Angle Conversion  IU=rad  OU=deg
  Dot Product{,1..6} (7 alike) : DotProduct  InputSameDT=on  OutDataTypeStr=Inherit: Inherit via internal rule
  DynamicPressure : Subsystem
  Gain : Gain
  Gain1 : Gain  Gain=MAC3
  Gain4 : Gain
  Trigonometric Function2 : Trigonometry
  Trigonometric Function3 : Trigonometry  Operator=cos
  wing : Subsystem
  FzR : Outport
  FxR : Outport  Port=2
  MacR : Outport  Port=3
  wires:
  wing/3(cm) -> Gain1/1
  Gain4/1 -> Dot Product1/1
  Gain/1 -> Dot Product/1
  wing/1(cl) -> Gain/1
  v/1 -> DynamicPressure/1(v), wing/3(airspeed)
  delta_R/1 -> wing/2(Delta)
  DynamicPressure/1(p) -> Dot Product/2, Dot Product1/2, Dot Product2/2
  wing/2(cd) -> Gain4/1
  Gain1/1 -> Dot Product2/1
  Dot Product2/1 -> MacR/1
  Angle Conversion/1 -> wing/1(Alpha)
  Trigonometric Function2/1 -> [sin]
  "ALFA "/1 -> Trigonometric Function2/1, Trigonometric Function3/1, Angle Conversion/1
  Trigonometric Function3/1 -> [cos]
  Dot Product/1 -> [L]
  Dot Product1/1 -> [D]
  [L] -> Dot Product3/1
  [cos] -> Dot Product3/2
  [D] -> Dot Product4/1
  [sin] -> Dot Product4/2
  Dot Product3/1 -> Add/1
  Dot Product4/1 -> Add/2
  Add/1 -> FzR/1
  [L] -> Dot Product5/1
  [sin] -> Dot Product5/2
  [D] -> Dot Product6/1
  [cos] -> Dot Product6/2
  Dot Product5/1 -> Add1/1
  Dot Product6/1 -> Add1/2
  Add1/1 -> FxR/1

== system TBS_SIM_UDP_HIL/Caipriha Airframe2/Aerodynamic Coefficient/Segment1/right wing/DynamicPressure&area ==
  v : Inport
  Gain1 : Gain  Gain=air_density
  Gain2 : Gain  Gain=0.5
  Gain3 : Gain  Gain=S_seg1*2
  Math Function : Math  Operator=magnitude^2  SaturateOnIntegerOverflow=on
  p : Outport
  wires:
  Gain3/1 -> p/1
  Gain2/1 -> Gain3/1
  Gain1/1 -> Gain2/1
  Math Function/1 -> Gain1/1
  v/1 -> Math Function/1

== system TBS_SIM_UDP_HIL/Caipriha Airframe2/Aerodynamic Coefficient/Segment1/right wing/wing ==
  Alpha : Inport
  Delta : Inport  Port=2
  airspeed : Inport  Port=3
  AirspeedLookup : PreLookup  BreakpointsData=as  BeginIndexSearchUsingPreviousIndexResult=on  ExtrapMethod=Linear
  AlphaLookup : PreLookup  BreakpointsData=alpha_vec_0  BeginIndexSearchUsingPreviousIndexResult=on  ExtrapMethod=Linear
  CD : Interpolation_n-D  NumberOfTableDimensions=3  Table=ORIGIN_CD  ExtrapMethod=Clip  DiagnosticForOutOfRangeInput=Warning  InternalRulePriority=Speed
      settings: InputPortMap=u0,u1,u2,u3,u4,u5
  CD1 : Interpolation_n-D  NumberOfTableDimensions=3  Table=ORIGIN_CM  ExtrapMethod=Clip  DiagnosticForOutOfRangeInput=Warning  InternalRulePriority=Speed
      settings: InputPortMap=u0,u1,u2,u3,u4,u5
  CL : Interpolation_n-D  NumberOfTableDimensions=3  Table=ORIGIN_CL  ExtrapMethod=Clip  DiagnosticForOutOfRangeInput=Warning  InternalRulePriority=Speed
      settings: InputPortMap=u0,u1,u2,u3,u4,u5
  DeltaLookup : PreLookup  BreakpointsData=ORIGIN_DELTA  BeginIndexSearchUsingPreviousIndexResult=on  ExtrapMethod=Linear
  cl : Outport
  cd : Outport  Port=2
  cm : Outport  Port=3
  wires:
  Alpha/1 -> AlphaLookup/1
  airspeed/1 -> AirspeedLookup/1
  DeltaLookup/1 -> CD1/5, CL/5, CD/5
  DeltaLookup/2 -> CD1/6, CL/6, CD/6
  CL/1 -> cl/1
  AirspeedLookup/1 -> CD1/1, CD/1, CL/1
  AirspeedLookup/2 -> CD1/2, CD/2, CL/2
  AlphaLookup/1 -> CD/3, CD1/3, CL/3
  AlphaLookup/2 -> CD1/4, CD/4, CL/4
  CD/1 -> cd/1
  CD1/1 -> cm/1
  Delta/1 -> DeltaLookup/1

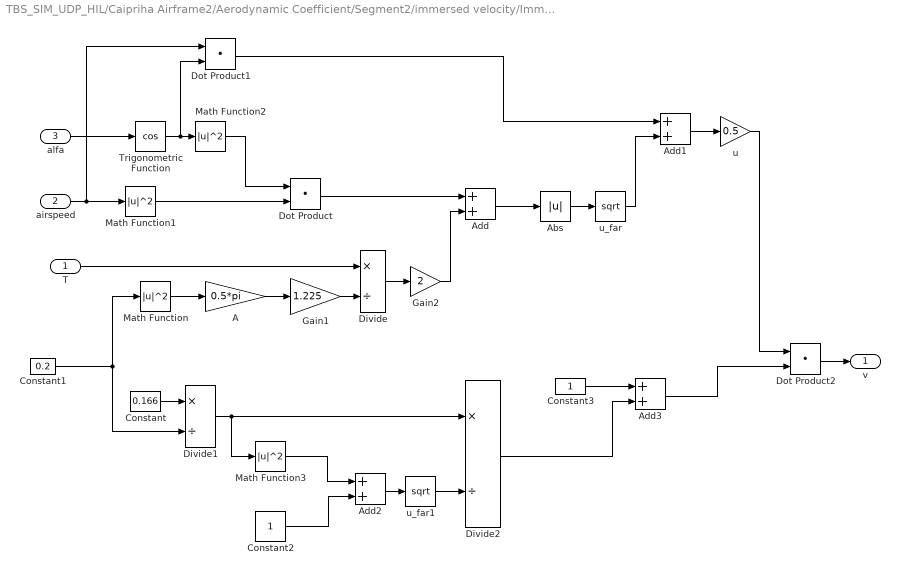
== system TBS_SIM_UDP_HIL/Caipriha Airframe2/Aerodynamic Coefficient/Segment2/immersed velocity/Immersed velocity  ==
  T : Inport
  airspeed : Inport  Port=2
  alfa : Inport  Port=3
  A : Gain  Gain=0.5*pi
  Abs : Abs
  Add{,1..3} (4 alike) : Sum
  Constant : Constant  Value=0.166
  Constant1 : Constant  Value=0.2
  Constant2 : Constant
  Constant3 : Constant
  Divide : Product  Inputs=*/
  Divide1 : Product  Inputs=*/
  Divide2 : Product  Inputs=*/
  Dot Product : DotProduct  InputSameDT=on  OutDataTypeStr=Inherit: Inherit via internal rule
  Dot Product1 : DotProduct  InputSameDT=on  OutDataTypeStr=Inherit: Inherit via internal rule
  Dot Product2 : DotProduct  InputSameDT=on  OutDataTypeStr=Inherit: Inherit via internal rule
  Gain1 : Gain  Gain=1.225
  Gain2 : Gain  Gain=2
  Math Function{,1..3} (4 alike) : Math  Operator=magnitude^2  SaturateOnIntegerOverflow=on
  Trigonometric Function : Trigonometry  Operator=cos
  u : Gain  Gain=0.5
  u_far : Sqrt  SaturateOnIntegerOverflow=on
  u_far1 : Sqrt  SaturateOnIntegerOverflow=on
  v : Outport
  wires:
  Add3/1 -> Dot Product2/2
  Divide2/1 -> Add3/2
  u/1 -> Dot Product2/1
  Constant3/1 -> Add3/1
  Divide1/1 -> Divide2/1, Math Function3/1
  u_far1/1 -> Divide2/2
  Add2/1 -> u_far1/1
  Constant2/1 -> Add2/2
  Math Function3/1 -> Add2/1
  Constant/1 -> Divide1/1
  Add1/1 -> u/1
  Dot Product1/1 -> Add1/1
  u_far/1 -> Add1/2
  Math Function2/1 -> Dot Product/1
  Trigonometric Function/1 -> Math Function2/1, Dot Product1/2
  Abs/1 -> u_far/1
  Add/1 -> Abs/1
  Gain2/1 -> Add/2
  Dot Product/1 -> Add/1
  Math Function1/1 -> Dot Product/2
  alfa/1 -> Trigonometric Function/1
  airspeed/1 -> Math Function1/1, Dot Product1/1
  Divide/1 -> Gain2/1
  T/1 -> Divide/1
  Gain1/1 -> Divide/2
  A/1 -> Gain1/1
  Math Function/1 -> A/1
  Constant1/1 -> Math Function/1, Divide1/2
  Dot Product2/1 -> v/1

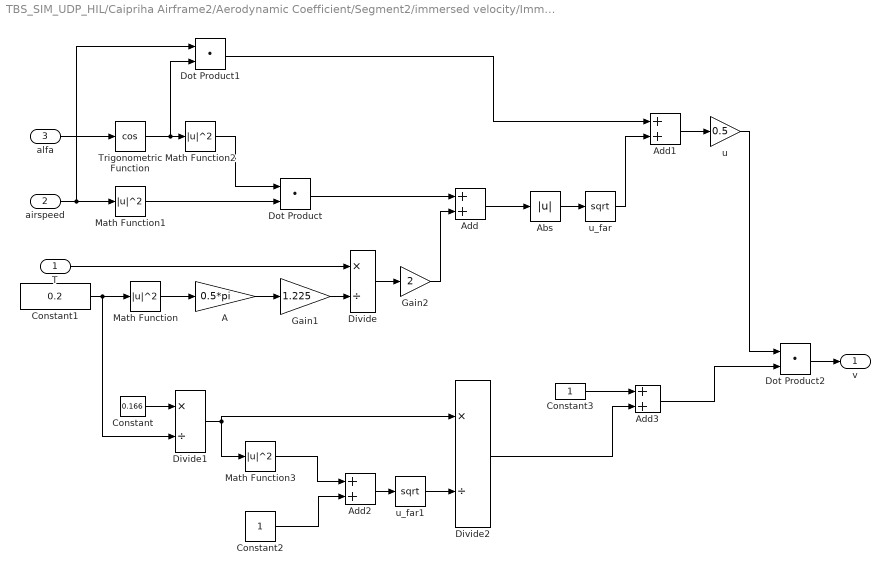
== system TBS_SIM_UDP_HIL/Caipriha Airframe2/Aerodynamic Coefficient/Segment2/immersed velocity/Immersed velocity 1 ==
  T : Inport
  airspeed : Inport  Port=2
  alfa : Inport  Port=3
  A : Gain  Gain=0.5*pi
  Abs : Abs
  Add{,1..3} (4 alike) : Sum
  Constant : Constant  Value=0.166
  Constant1 : Constant  Value=0.2
  Constant2 : Constant
  Constant3 : Constant
  Divide : Product  Inputs=*/
  Divide1 : Product  Inputs=*/
  Divide2 : Product  Inputs=*/
  Dot Product : DotProduct  InputSameDT=on  OutDataTypeStr=Inherit: Inherit via internal rule
  Dot Product1 : DotProduct  InputSameDT=on  OutDataTypeStr=Inherit: Inherit via internal rule
  Dot Product2 : DotProduct  InputSameDT=on  OutDataTypeStr=Inherit: Inherit via internal rule
  Gain1 : Gain  Gain=1.225
  Gain2 : Gain  Gain=2
  Math Function{,1..3} (4 alike) : Math  Operator=magnitude^2  SaturateOnIntegerOverflow=on
  Trigonometric Function : Trigonometry  Operator=cos
  u : Gain  Gain=0.5
  u_far : Sqrt  SaturateOnIntegerOverflow=on
  u_far1 : Sqrt  SaturateOnIntegerOverflow=on
  v : Outport
  wires:
  Add3/1 -> Dot Product2/2
  Divide2/1 -> Add3/2
  Constant3/1 -> Add3/1
  Dot Product2/1 -> v/1
  u/1 -> Dot Product2/1
  Divide1/1 -> Math Function3/1, Divide2/1
  u_far1/1 -> Divide2/2
  Add2/1 -> u_far1/1
  Constant2/1 -> Add2/2
  Math Function3/1 -> Add2/1
  Constant/1 -> Divide1/1
  Add1/1 -> u/1
  Dot Product1/1 -> Add1/1
  u_far/1 -> Add1/2
  Math Function2/1 -> Dot Product/1
  Trigonometric Function/1 -> Math Function2/1, Dot Product1/2
  Abs/1 -> u_far/1
  Add/1 -> Abs/1
  Gain2/1 -> Add/2
  Dot Product/1 -> Add/1
  Math Function1/1 -> Dot Product/2
  alfa/1 -> Trigonometric Function/1
  airspeed/1 -> Math Function1/1, Dot Product1/1
  Divide/1 -> Gain2/1
  T/1 -> Divide/1
  Gain1/1 -> Divide/2
  A/1 -> Gain1/1
  Math Function/1 -> A/1
  Constant1/1 -> Math Function/1, Divide1/2

== system TBS_SIM_UDP_HIL/Caipriha Airframe2/Aerodynamic Coefficient/Segment2/left wing/DynamicPressure ==
  v : Inport
  Gain1 : Gain  Gain=air_density
  Gain2 : Gain  Gain=0.5
  Gain3 : Gain  Gain=S_seg2
  Math Function : Math  Operator=magnitude^2  SaturateOnIntegerOverflow=on
  p : Outport
  wires:
  Gain3/1 -> p/1
  Gain2/1 -> Gain3/1
  Gain1/1 -> Gain2/1
  Math Function/1 -> Gain1/1
  v/1 -> Math Function/1

== system TBS_SIM_UDP_HIL/Caipriha Airframe2/Aerodynamic Coefficient/Segment2/left wing/wing ==
  Alpha : Inport
  Delta : Inport  Port=2
  airspeed : Inport  Port=3
  AirspeedLookup : PreLookup  BreakpointsData=as  BeginIndexSearchUsingPreviousIndexResult=on  ExtrapMethod=Linear
  AlphaLookup : PreLookup  BreakpointsData=alpha_vec_0  BeginIndexSearchUsingPreviousIndexResult=on  ExtrapMethod=Linear
  CD : Interpolation_n-D  NumberOfTableDimensions=3  Table=ORIGIN_CD  ExtrapMethod=Clip  DiagnosticForOutOfRangeInput=Warning  InternalRulePriority=Speed
      settings: InputPortMap=u0,u1,u2,u3,u4,u5
  CD1 : Interpolation_n-D  NumberOfTableDimensions=3  Table=ORIGIN_CM  ExtrapMethod=Clip  DiagnosticForOutOfRangeInput=Warning  InternalRulePriority=Speed
      settings: InputPortMap=u0,u1,u2,u3,u4,u5
  CL : Interpolation_n-D  NumberOfTableDimensions=3  Table=ORIGIN_CL  ExtrapMethod=Clip  DiagnosticForOutOfRangeInput=Warning  InternalRulePriority=Speed
      settings: InputPortMap=u0,u1,u2,u3,u4,u5
  DeltaLookup : PreLookup  BreakpointsData=ORIGIN_DELTA  BeginIndexSearchUsingPreviousIndexResult=on  ExtrapMethod=Linear
  cl : Outport
  cd : Outport  Port=2
  cm : Outport  Port=3
  wires:
  Alpha/1 -> AlphaLookup/1
  airspeed/1 -> AirspeedLookup/1
  DeltaLookup/1 -> CD1/5, CL/5, CD/5
  DeltaLookup/2 -> CD1/6, CL/6, CD/6
  CL/1 -> cl/1
  AirspeedLookup/1 -> CD1/1, CD/1, CL/1
  AirspeedLookup/2 -> CD1/2, CD/2, CL/2
  AlphaLookup/1 -> CD/3, CD1/3, CL/3
  AlphaLookup/2 -> CD1/4, CD/4, CL/4
  CD/1 -> cd/1
  CD1/1 -> cm/1
  Delta/1 -> DeltaLookup/1

== system TBS_SIM_UDP_HIL/Caipriha Airframe2/Aerodynamic Coefficient/Segment2/right wing/DynamicPressure ==
  v : Inport
  Gain1 : Gain  Gain=air_density
  Gain2 : Gain  Gain=0.5
  Gain3 : Gain  Gain=S_seg2
  Math Function : Math  Operator=magnitude^2  SaturateOnIntegerOverflow=on
  p : Outport
  wires:
  Gain3/1 -> p/1
  Gain2/1 -> Gain3/1
  Gain1/1 -> Gain2/1
  Math Function/1 -> Gain1/1
  v/1 -> Math Function/1

== system TBS_SIM_UDP_HIL/Caipriha Airframe2/Aerodynamic Coefficient/Segment2/right wing/wing ==
  Alpha : Inport
  Delta : Inport  Port=2
  airspeed : Inport  Port=3
  AirspeedLookup : PreLookup  BreakpointsData=as  BeginIndexSearchUsingPreviousIndexResult=on  ExtrapMethod=Linear
  AlphaLookup : PreLookup  BreakpointsData=alpha_vec_0  BeginIndexSearchUsingPreviousIndexResult=on  ExtrapMethod=Linear
  CD : Interpolation_n-D  NumberOfTableDimensions=3  Table=ORIGIN_CD  ExtrapMethod=Clip  DiagnosticForOutOfRangeInput=Warning  InternalRulePriority=Speed
      settings: InputPortMap=u0,u1,u2,u3,u4,u5
  CD1 : Interpolation_n-D  NumberOfTableDimensions=3  Table=ORIGIN_CM  ExtrapMethod=Clip  DiagnosticForOutOfRangeInput=Warning  InternalRulePriority=Speed
      settings: InputPortMap=u0,u1,u2,u3,u4,u5
  CL : Interpolation_n-D  NumberOfTableDimensions=3  Table=ORIGIN_CL  ExtrapMethod=Clip  DiagnosticForOutOfRangeInput=Warning  InternalRulePriority=Speed
      settings: InputPortMap=u0,u1,u2,u3,u4,u5
  DeltaLookup : PreLookup  BreakpointsData=ORIGIN_DELTA  BeginIndexSearchUsingPreviousIndexResult=on  ExtrapMethod=Linear
  cl : Outport
  cd : Outport  Port=2
  cm : Outport  Port=3
  wires:
  Alpha/1 -> AlphaLookup/1
  airspeed/1 -> AirspeedLookup/1
  DeltaLookup/1 -> CD1/5, CL/5, CD/5
  DeltaLookup/2 -> CD1/6, CL/6, CD/6
  CL/1 -> cl/1
  AirspeedLookup/1 -> CD1/1, CD/1, CL/1
  AirspeedLookup/2 -> CD1/2, CD/2, CL/2
  AlphaLookup/1 -> CD/3, CD1/3, CL/3
  AlphaLookup/2 -> CD1/4, CD/4, CL/4
  CD/1 -> cd/1
  CD1/1 -> cm/1
  Delta/1 -> DeltaLookup/1

== system TBS_SIM_UDP_HIL/Caipriha Airframe2/Aerodynamic Coefficient/Segment3L1/wing/DynamicPressure ==
  v : Inport
  Gain1 : Gain  Gain=air_density
  Gain2 : Gain  Gain=0.5
  Gain3 : Gain  Gain=S_seg3
  Math Function : Math  Operator=magnitude^2  SaturateOnIntegerOverflow=on
  p : Outport
  wires:
  Gain3/1 -> p/1
  Gain2/1 -> Gain3/1
  Gain1/1 -> Gain2/1
  Math Function/1 -> Gain1/1
  v/1 -> Math Function/1

== system TBS_SIM_UDP_HIL/Caipriha Airframe2/Aerodynamic Coefficient/Segment3L1/wing/wing ==
  Alpha : Inport
  Delta : Inport  Port=2
  airspeed : Inport  Port=3
  AirspeedLookup : PreLookup  BreakpointsData=as  BeginIndexSearchUsingPreviousIndexResult=on  ExtrapMethod=Linear
  AlphaLookup : PreLookup  BreakpointsData=alpha_vec_0  BeginIndexSearchUsingPreviousIndexResult=on  ExtrapMethod=Linear
  CD : Interpolation_n-D  NumberOfTableDimensions=3  Table=ORIGIN_CD  ExtrapMethod=Clip  DiagnosticForOutOfRangeInput=Warning  InternalRulePriority=Speed
      settings: InputPortMap=u0,u1,u2,u3,u4,u5
  CD1 : Interpolation_n-D  NumberOfTableDimensions=3  Table=ORIGIN_CM  ExtrapMethod=Clip  DiagnosticForOutOfRangeInput=Warning  InternalRulePriority=Speed
      settings: InputPortMap=u0,u1,u2,u3,u4,u5
  CL : Interpolation_n-D  NumberOfTableDimensions=3  Table=ORIGIN_CL  ExtrapMethod=Clip  DiagnosticForOutOfRangeInput=Warning  InternalRulePriority=Speed
      settings: InputPortMap=u0,u1,u2,u3,u4,u5
  DeltaLookup : PreLookup  BreakpointsData=ORIGIN_DELTA  BeginIndexSearchUsingPreviousIndexResult=on  ExtrapMethod=Linear
  cl : Outport
  cd : Outport  Port=2
  cm : Outport  Port=3
  wires:
  Alpha/1 -> AlphaLookup/1
  airspeed/1 -> AirspeedLookup/1
  DeltaLookup/1 -> CD1/5, CL/5, CD/5
  DeltaLookup/2 -> CD1/6, CL/6, CD/6
  CL/1 -> cl/1
  AirspeedLookup/1 -> CD1/1, CD/1, CL/1
  AirspeedLookup/2 -> CD1/2, CD/2, CL/2
  AlphaLookup/1 -> CD/3, CD1/3, CL/3
  AlphaLookup/2 -> CD1/4, CD/4, CL/4
  CD/1 -> cd/1
  CD1/1 -> cm/1
  Delta/1 -> DeltaLookup/1

== system TBS_SIM_UDP_HIL/Caipriha Airframe2/Aerodynamic Coefficient/Segment3R/right wing/DynamicPressure ==
  v : Inport
  Gain1 : Gain  Gain=air_density
  Gain2 : Gain  Gain=0.5
  Gain3 : Gain  Gain=S_seg3
  Math Function : Math  Operator=magnitude^2  SaturateOnIntegerOverflow=on
  p : Outport
  wires:
  Gain3/1 -> p/1
  Gain2/1 -> Gain3/1
  Gain1/1 -> Gain2/1
  Math Function/1 -> Gain1/1
  v/1 -> Math Function/1

== system TBS_SIM_UDP_HIL/Caipriha Airframe2/Aerodynamic Coefficient/Segment3R/right wing/wing ==
  Alpha : Inport
  Delta : Inport  Port=2
  airspeed : Inport  Port=3
  AirspeedLookup : PreLookup  BreakpointsData=as  BeginIndexSearchUsingPreviousIndexResult=on  ExtrapMethod=Linear
  AlphaLookup : PreLookup  BreakpointsData=alpha_vec_0  BeginIndexSearchUsingPreviousIndexResult=on  ExtrapMethod=Linear
  CD : Interpolation_n-D  NumberOfTableDimensions=3  Table=ORIGIN_CD  ExtrapMethod=Clip  DiagnosticForOutOfRangeInput=Warning  InternalRulePriority=Speed
      settings: InputPortMap=u0,u1,u2,u3,u4,u5
  CD1 : Interpolation_n-D  NumberOfTableDimensions=3  Table=ORIGIN_CM  ExtrapMethod=Clip  DiagnosticForOutOfRangeInput=Warning  InternalRulePriority=Speed
      settings: InputPortMap=u0,u1,u2,u3,u4,u5
  CL : Interpolation_n-D  NumberOfTableDimensions=3  Table=ORIGIN_CL  ExtrapMethod=Clip  DiagnosticForOutOfRangeInput=Warning  InternalRulePriority=Speed
      settings: InputPortMap=u0,u1,u2,u3,u4,u5
  DeltaLookup : PreLookup  BreakpointsData=ORIGIN_DELTA  BeginIndexSearchUsingPreviousIndexResult=on  ExtrapMethod=Linear
  cl : Outport
  cd : Outport  Port=2
  cm : Outport  Port=3
  wires:
  Alpha/1 -> AlphaLookup/1
  airspeed/1 -> AirspeedLookup/1
  DeltaLookup/1 -> CD1/5, CL/5, CD/5
  DeltaLookup/2 -> CD1/6, CL/6, CD/6
  CL/1 -> cl/1
  AirspeedLookup/1 -> CD1/1, CD/1, CL/1
  AirspeedLookup/2 -> CD1/2, CD/2, CL/2
  AlphaLookup/1 -> CD/3, CD1/3, CL/3
  AlphaLookup/2 -> CD1/4, CD/4, CL/4
  CD/1 -> cd/1
  CD1/1 -> cm/1
  Delta/1 -> DeltaLookup/1
